simulink model "problem7"  (R2020b)
settings: Solver=VariableStepAuto  StartTime=0.0  StopTime=10.0  RelTol=1e-3
settings Model: Creator=adity  LastModifiedBy=adity

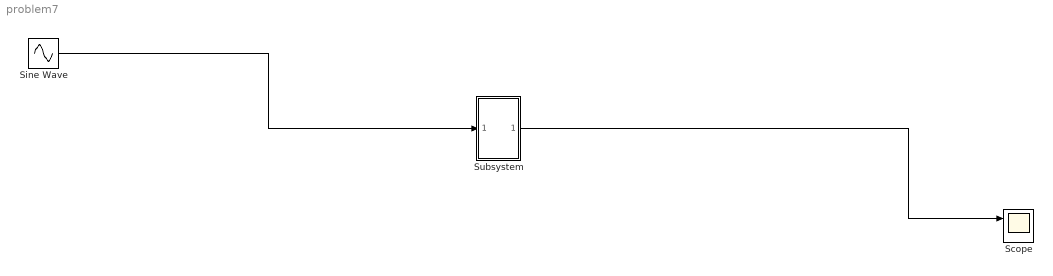
== system problem7 ==
  Scope : Scope  NumInputPorts=2
  Sine Wave : Sin  SampleTime=0
  Subsystem : Subsystem
  wires:
  Sine Wave/1 -> Subsystem/1(In1)
  Subsystem/1(Out1) -> Scope/1

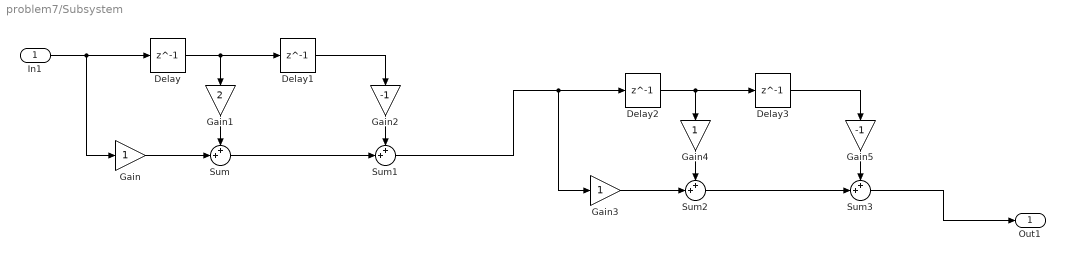
== system problem7/Subsystem ==
  In1 : Inport
  Delay{,1..3} (4 alike) : Delay  DelayLength=1
  Gain : Gain
  Gain1 : Gain  Gain=2
  Gain2 : Gain  Gain=-1
  Gain3 : Gain
  Gain4 : Gain
  Gain5 : Gain  Gain=-1
  Sum{,1..3} (4 alike) : Sum  Inputs=++|
  Out1 : Outport
  wires:
  Delay/1 -> Gain1/1, Delay1/1
  Gain5/1 -> Sum3/1
  Gain3/1 -> Sum2/2
  Sum1/1 -> Gain3/1, Delay2/1
  Delay1/1 -> Gain2/1
  Sum2/1 -> Sum3/2
  Sum/1 -> Sum1/2
  In1/1 -> Gain/1, Delay/1
  Delay2/1 -> Gain4/1, Delay3/1
  Gain/1 -> Sum/2
  Delay3/1 -> Gain5/1
  Gain1/1 -> Sum/1
  Gain2/1 -> Sum1/1
  Gain4/1 -> Sum2/1
  Sum3/1 -> Out1/1
